simulink model "Final_Q1_B_end"  (R2019a)
settings: Solver=VariableStepAuto  StartTime=0.0  StopTime=60.0  RelTol=1e-3
settings Model: SimulationMode=accelerator  Creator=kullanıcı  LastModifiedBy=hp

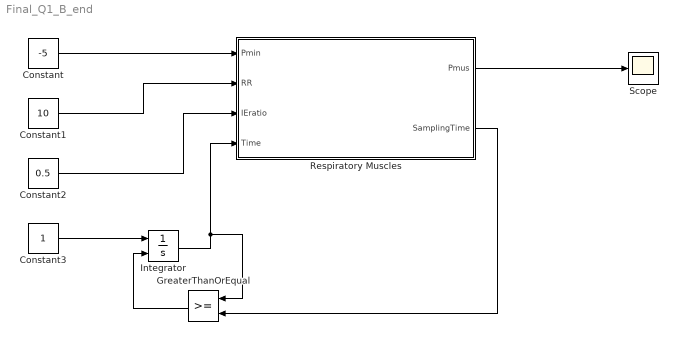
== system Final_Q1_B_end ==
  Constant : Constant  Value=-5
  Constant1 : Constant  Value=10
  Constant2 : Constant  Value=0.5
  Constant3 : Constant
  GreaterThanOrEqual : RelationalOperator  OutDataTypeStr=boolean  RndMeth=Simplest
  Integrator : Integrator  ExternalReset=rising
  Respiratory Muscles : MATLAB Function  TreatAsAtomicUnit=on
  Scope : Scope
  wires:
  Constant/1 -> Respiratory Muscles/1(Pmin)
  Constant1/1 -> Respiratory Muscles/2(RR)
  Constant2/1 -> Respiratory Muscles/3(IEratio)
  Constant3/1 -> Integrator/1
  GreaterThanOrEqual/1 -> Integrator/2
  Integrator/1 -> Respiratory Muscles/4(Time), GreaterThanOrEqual/1
  Respiratory Muscles/2(SamplingTime) -> GreaterThanOrEqual/2
  Respiratory Muscles/1(Pmus) -> Scope/1

== matlab function Final_Q1_B_end/Respiratory Muscles ==
  data: Pmin input; Pmus output; RR input; IEratio input; Time input; SamplingTime output
function [Pmus,SamplingTime] = fcn(Pmin,RR ,IEratio, Time)
T = 60/RR;
SamplingTime = T; 
TE = T/(1 + IEratio);
TI = T - TE;
Tau = TE / 10;

if (Time <= TI)

    Pmus = Pmin*(1/(TI*TE))*(T*Time -Time^2)
    

else 
    
    Pmus = (Pmin/(1 - exp((-TE/Tau))))*(exp(((Time - TI)/(-Tau)))-exp(((-TE)/(Tau))))
end


end
